simulink model "SoftwareArchitecture"  (R2020a)
settings: Solver=VariableStepAuto  StartTime=0.0  StopTime=10.0  RelTol=1e-3
settings Model: Creator=pav4609  LastModifiedBy=pav4609

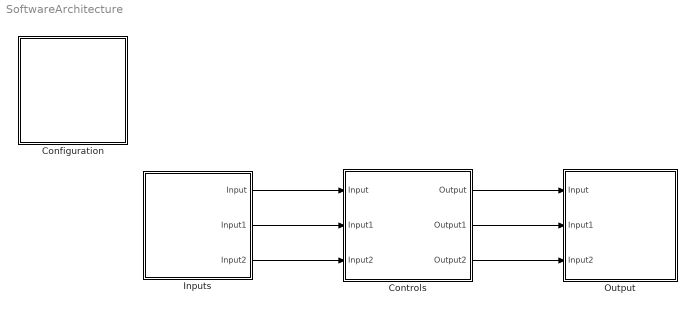
== system SoftwareArchitecture ==
  Configuration : Subsystem
  Controls : Subsystem
  Inputs : Subsystem
  Output : Subsystem
  wires:
  Inputs/3(Input2) -> Controls/3(Input2)
  Inputs/2(Input1) -> Controls/2(Input1)
  Inputs/1(Input) -> Controls/1(Input)
  Controls/1(Output) -> Output/1(Input)
  Controls/2(Output1) -> Output/2(Input1)
  Controls/3(Output2) -> Output/3(Input2)

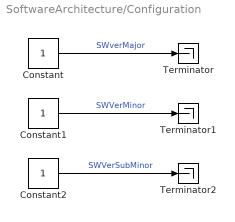
== system SoftwareArchitecture/Configuration ==
  Constant : Constant
  Constant1 : Constant
  Constant2 : Constant
  Terminator : Terminator
  Terminator1 : Terminator
  Terminator2 : Terminator
  wires:
  Constant/1 -> Terminator/1  "SWverMajor"
  Constant1/1 -> Terminator1/1  "SWVerMinor"
  Constant2/1 -> Terminator2/1  "SWVerSubMinor"

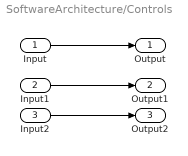
== system SoftwareArchitecture/Controls ==
  Input : Inport
  Input1 : Inport  Port=2
  Input2 : Inport  Port=3
  Output : Outport
  Output1 : Outport  Port=2
  Output2 : Outport  Port=3
  wires:
  Input2/1 -> Output2/1
  Input1/1 -> Output1/1
  Input/1 -> Output/1

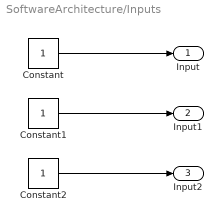
== system SoftwareArchitecture/Inputs ==
  Constant : Constant
  Constant1 : Constant
  Constant2 : Constant
  Input : Outport
  Input1 : Outport  Port=2
  Input2 : Outport  Port=3
  wires:
  Constant/1 -> Input/1
  Constant1/1 -> Input1/1
  Constant2/1 -> Input2/1

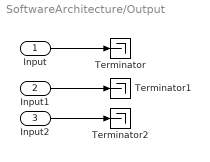
== system SoftwareArchitecture/Output ==
  Input : Inport
  Input1 : Inport  Port=2
  Input2 : Inport  Port=3
  Terminator : Terminator
  Terminator1 : Terminator
  Terminator2 : Terminator
  wires:
  Input2/1 -> Terminator2/1
  Input1/1 -> Terminator1/1
  Input/1 -> Terminator/1
